simulink library "FancyGravity"  (R2020b)
settings: Solver=VariableStepAuto  StartTime=0.0  StopTime=10.0  RelTol=1e-3
libraries: aerolibgravity2 x3, aerolibtransform2 x1
settings Model: Creator=dbell44  LastModifiedBy=dbell44

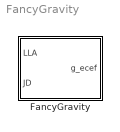
== system FancyGravity ==
  FancyGravity : Subsystem

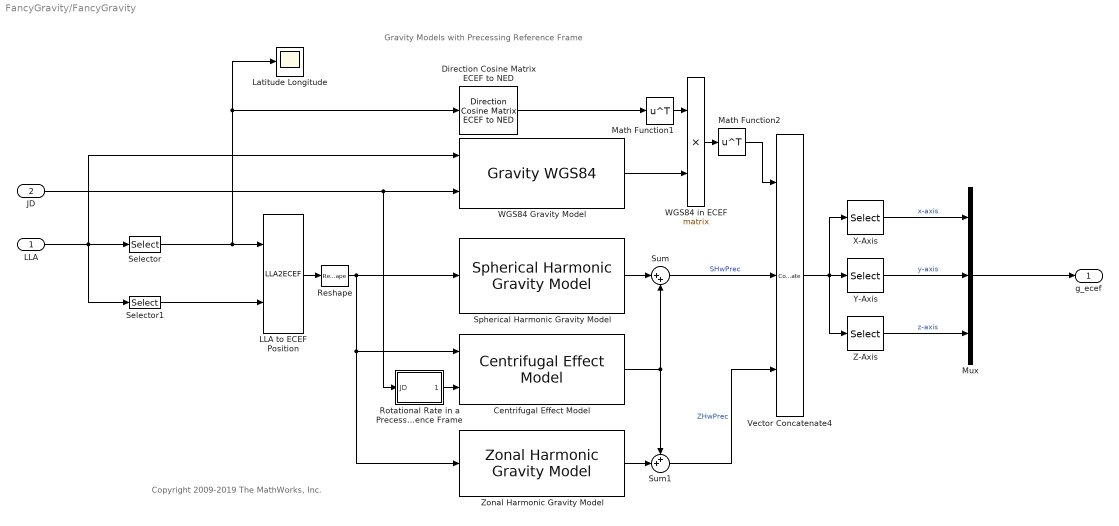
== system FancyGravity/FancyGravity ==
  note: Copyright 2009-2019 The MathWorks, Inc.
  note: Gravity Models with Precessing Reference Frame
  LLA : Inport
  JD : Inport  Port=2
  Centrifugal Effect Model : aerolibgravity2/Centrifugal Effect Model  ptype=Custom  omega=7.2921150e-005  rate_loc=on
      settings: SourceProductName=Aerospace Blockset
  Direction Cosine Matrix ECEF to NED : aerolibtransform2/Direction Cosine Matrix ECEF to NED
      settings: SourceProductName=Aerospace Blockset
  LLA to ECEF Position : LLA2ECEF  R=6378137
  Latitude Longitude : Scope
  Math Function1 : Math  Operator=transpose  SignedPower=on  SaturateOnIntegerOverflow=on
  Math Function2 : Math  Operator=transpose  SignedPower=on  SaturateOnIntegerOverflow=on
  Mux : Mux  Inputs=3
  Reshape : Reshape  OutputDimensionality=Row vector (2-D)
  Rotational Rate in a Precessing Reference Frame : Subsystem
  Selector : Selector  InputPortWidth=3  IndexOptions=Index vector (dialog)  Indices=[1 2]  OutputSizes=1
  Selector1 : Selector  InputPortWidth=3  IndexOptions=Index vector (dialog)  Indices=[3]  OutputSizes=1
  Spherical Harmonic Gravity Model : aerolibgravity2/Spherical Harmonic Gravity Model  units=Metric (MKS)  degree=120  action=Warning  ptype=EGM2008  datafile='aerogmm2b'
      settings: SourceProductName=Aerospace Blockset
  Sum : Sum  Inputs=|++
  Sum1 : Sum  Inputs=++|
  Vector Concatenate4 : Concatenate  NumInputs=3  Mode=Multidimensional array
  WGS84 in ECEF : Product  Multiplication=Matrix(*)  RndMeth=Zero
  "WGS84 Gravity Model  " : GravityWGS84  model=WGS84 Exact  jd_loc=on  no_centrifugal=off  action=None
  X-Axis : Selector  NumberOfDimensions=2  IndexMode=Zero-based  InputPortWidth=3  IndexOptions=Index vector (dialog),Index vector (dialog)  Indices=0,0  OutputSizes=1,1
  Y-Axis : Selector  NumberOfDimensions=2  IndexMode=Zero-based  InputPortWidth=3  IndexOptions=Index vector (dialog),Index vector (dialog)  Indices=1,1  OutputSizes=1,1
  Z-Axis : Selector  NumberOfDimensions=2  IndexMode=Zero-based  InputPortWidth=3  IndexOptions=Index vector (dialog),Index vector (dialog)  Indices=2,2  OutputSizes=1,1
  Zonal Harmonic Gravity Model : aerolibgravity2/Zonal Harmonic Gravity Model  units=Metric (MKS)  degree=4  action=Warning  ptype=Earth  R=6378136.3  GM=398600441500000  jvalue=[1.0826269e-03 -2.5323000e-06 -1.6204000e-06]
      settings: SourceProductName=Aerospace Blockset
  g_ecef : Outport
  wires:
  Zonal Harmonic Gravity Model/1 -> Sum1/2
  Math Function1/1 -> WGS84 in ECEF/1
  Sum1/1 -> Vector Concatenate4/3  "ZHwPrec"
  Math Function2/1 -> Vector Concatenate4/1
  Spherical Harmonic Gravity Model/1 -> Sum/1
  Selector/1 -> Direction Cosine Matrix ECEF to NED/1, Latitude Longitude/1, LLA to ECEF Position/1
  LLA/1 -> "WGS84 Gravity Model  "/1, Selector1/1, Selector/1
  Sum/1 -> Vector Concatenate4/2  "SHwPrec"
  Reshape/1 -> Zonal Harmonic Gravity Model/1, Centrifugal Effect Model/1, Spherical Harmonic Gravity Model/1
  Centrifugal Effect Model/1 -> Sum/2, Sum1/1
  Direction Cosine Matrix ECEF to NED/1 -> Math Function1/1
  Selector1/1 -> LLA to ECEF Position/2
  LLA to ECEF Position/1 -> Reshape/1
  WGS84 in ECEF/1 -> Math Function2/1
  JD/1 -> "WGS84 Gravity Model  "/2, Rotational Rate in a Precessing Reference Frame/1(JD)
  "WGS84 Gravity Model  "/1 -> WGS84 in ECEF/2
  Rotational Rate in a Precessing Reference Frame/1(omega) -> Centrifugal Effect Model/2
  X-Axis/1 -> Mux/1  "x-axis"
  Y-Axis/1 -> Mux/2  "y-axis"
  Vector Concatenate4/1 -> Y-Axis/1, X-Axis/1, Z-Axis/1
  Z-Axis/1 -> Mux/3  "z-axis"
  Mux/1 -> g_ecef/1

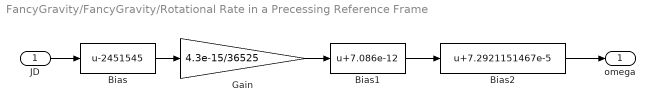
== system FancyGravity/FancyGravity/Rotational Rate in a Precessing Reference Frame ==
  JD : Inport
  Bias : Bias  Bias=-2451545
  Bias1 : Bias  Bias=7.086e-12
  Bias2 : Bias  Bias=7.2921151467e-5
  Gain : Gain  Gain=4.3e-15/36525
  omega : Outport  VectorParamsAs1DForOutWhenUnconnected=off
  wires:
  JD/1 -> Bias/1
  Bias/1 -> Gain/1
  Gain/1 -> Bias1/1
  Bias1/1 -> Bias2/1
  Bias2/1 -> omega/1
